simulink model "Model_Platform"  (R2018a)
settings: Solver=ode1  StartTime=0.0  StopTime=inf  FixedStep=0.001  RelTol=1e-3  EnableMultiTasking=on
PreLoadFcn:
  | ;HLABlocksetInit;;HLABlocksetInit;;HLABlocksetInit;
PostLoadFcn:
  | ;set_param(gcs,'PostCodeGenCommand', 'rtw_defines(buildInfo)');;set_param(gcs,'PostCodeGenCommand', 'rtw_defines(buildInfo)');;set_param(gcs,'PostCodeGenCommand', 'rtw_defines(buildInfo)');
undefined symbols (not defined in the file or in its folder): eng_speed, Heading_init, inertiaLateral, Joystick, Newton, omega_engine, omega_max, omega_wheel, Para, radiusWheel, Raphson, Standard_Devices, torque, Torque_lost, Torque_lost_wheel, X_init, Y_init, Z_init
libraries: simulink x26, dspnetwork x4, rtwinlib x2, PC_Simulator_Lib x2, vrlib x1
(part 3 of 4)

== system Model_Platform/Vehicle model/Drive_Train/4_Wheels_drive_train_and_Brake/Brake/Subsystem ==
  Torque_Brake_Nm : Inport
  Omega_rad/s : Inport  Port=2
  Compare To Constant : simulink/Logic and Bit Operations/Compare To Constant  relop=>=  const=0.1  OutDataTypeStr=uint8
  Compare To Constant1 : simulink/Logic and Bit Operations/Compare To Constant  relop=<=  const=-0.1  OutDataTypeStr=uint8
  Data Type Conversion : DataTypeConversion
  Logical Operator : Logic  Operator=OR  AllPortsSameDT=off  OutDataTypeStr=boolean
  Product : Product  Inputs=3  RndMeth=Zero
  Rate Limiter1 : RateLimiter  SampleTimeMode=inherited
  Sign : Signum
  Torque_Brake_act_Nm : Outport
  wires:
  Torque_Brake_Nm/1 -> Product/1
  Omega_rad/s/1 -> Compare To Constant1/1, Compare To Constant/1, Sign/1
  Product/1 -> Torque_Brake_act_Nm/1
  Sign/1 -> Product/2
  Compare To Constant/1 -> Logical Operator/1
  Data Type Conversion/1 -> Rate Limiter1/1
  Logical Operator/1 -> Data Type Conversion/1
  Compare To Constant1/1 -> Logical Operator/2
  Rate Limiter1/1 -> Product/3

== system Model_Platform/Vehicle model/Drive_Train/4_Wheels_drive_train_and_Brake/Brake/Subsystem1 ==
  v_X_CoG[m|s] : Inport
  Brake_Pedal[norm] : Inport  Port=2
  Compare To Constant : simulink/Logic and Bit Operations/Compare To Constant  relop=<  const=0.7  OutDataTypeStr=uint8
  Compare To Constant1 : simulink/Logic and Bit Operations/Compare To Constant  relop=>  const=-1  OutDataTypeStr=uint8
  Compare To Constant2 : simulink/Logic and Bit Operations/Compare To Constant  relop=>=  const=0.01  OutDataTypeStr=uint8
  Compare To Constant3 : simulink/Logic and Bit Operations/Compare To Constant  relop=<  const=-0.1  OutDataTypeStr=uint8
  Constant : Constant  Value=0
  Constant1 : Constant  Value=3.5
  Constant2 : Constant
  Data Type Conversion : DataTypeConversion
  Gain1 : Gain  Gain=-100
  Logical Operator : Logic  Inputs=3  AllPortsSameDT=off  OutDataTypeStr=boolean
  Logical Operator1 : Logic  AllPortsSameDT=off  OutDataTypeStr=boolean
  Product : Product  Inputs=3
  Subtract : Sum  Inputs=+-
  Switch : Switch  Criteria=u2 > Threshold
  Out1 : Outport
  wires:
  Constant2/1 -> Switch/3
  Switch/1 -> Product/3
  Constant1/1 -> Switch/1
  Logical Operator1/1 -> Switch/2
  Compare To Constant3/1 -> Logical Operator1/2
  Brake_Pedal[norm]/1 -> Compare To Constant2/1
  Compare To Constant2/1 -> Logical Operator/3
  Data Type Conversion/1 -> Product/2
  Logical Operator/1 -> Data Type Conversion/1
  Compare To Constant1/1 -> Logical Operator/2, Logical Operator1/1
  Compare To Constant/1 -> Logical Operator/1
  Product/1 -> Out1/1
  Gain1/1 -> Product/1
  Subtract/1 -> Gain1/1
  Constant/1 -> Subtract/1
  v_X_CoG[m|s]/1 -> Subtract/2, Compare To Constant/1, Compare To Constant1/1, Compare To Constant3/1

== system Model_Platform/Vehicle model/Drive_Train/4_Wheels_drive_train_and_Brake/FL/Alpha_Kappa_Selector2 ==
  Vx : Inport
  Vy : Inport  Port=2
  omega : Inport  Port=3
  Rdyn : Inport  Port=4
  Fx : Inport  Port=5
  Dynamik Anteil2 : Subsystem
  Saturation : Saturate  UpperLimit=1  LowerLimit=-1
  alpha_calc : Subsystem
  kappa : Outport
  alpha : Outport  Port=2
  wires:
  Vy/1 -> alpha_calc/1(Vy)
  Vx/1 -> Dynamik Anteil2/2(Vx), alpha_calc/2(Vx)
  alpha_calc/1(alpha) -> alpha/1
  omega/1 -> Dynamik Anteil2/3(omega)
  Rdyn/1 -> Dynamik Anteil2/4(R)
  Saturation/1 -> kappa/1
  Dynamik Anteil2/1(k) -> Saturation/1
  Fx/1 -> Dynamik Anteil2/1(Fx)

== system Model_Platform/Vehicle model/Drive_Train/4_Wheels_drive_train_and_Brake/FL/Wheel dynamics ==
  F_x : Inport
  Torque_Drive_Nm : Inport  Port=2
  Torque_Brake_Nm : Inport  Port=3
  Add : Sum  Inputs=++--
  Friction : Subsystem
  Gain : Gain  Gain=radiusWheel
  Gain1 : Gain  Gain=-1
  Gain2 : Gain  Gain=1/(inertiaLateral/2)
  Integrator : Integrator
  Subsystem : Subsystem
  Terminator : Terminator
  omega_radPs : Outport
  omegaDot_radPs2 : Outport  Port=2
  wires:
  Subsystem/1(Torque_Brake_act_Nm) -> Terminator/1
  Torque_Brake_Nm/1 -> Add/4, Subsystem/1(Torque_Brake_Nm)
  Friction/1(Torque_friction) -> Add/3
  Integrator/1 -> Subsystem/2(Omega_rad/s), Friction/1(omega_radPs), omega_radPs/1
  Gain2/1 -> omegaDot_radPs2/1, Integrator/1
  Add/1 -> Gain2/1
  Torque_Drive_Nm/1 -> Add/2
  Gain1/1 -> Add/1
  F_x/1 -> Gain/1
  Gain/1 -> Gain1/1

== system Model_Platform/Vehicle model/Drive_Train/4_Wheels_drive_train_and_Brake/FR/Alpha_Kappa_Selector2 ==
  Vx : Inport
  Vy : Inport  Port=2
  omega : Inport  Port=3
  Rdyn : Inport  Port=4
  Fx : Inport  Port=5
  Dynamik Anteil2 : Subsystem
  Saturation : Saturate  UpperLimit=1  LowerLimit=-1
  alpha_calc : Subsystem
  kappa : Outport
  alpha : Outport  Port=2
  wires:
  Vy/1 -> alpha_calc/1(Vy)
  Vx/1 -> Dynamik Anteil2/2(Vx), alpha_calc/2(Vx)
  alpha_calc/1(alpha) -> alpha/1
  omega/1 -> Dynamik Anteil2/3(omega)
  Rdyn/1 -> Dynamik Anteil2/4(R)
  Saturation/1 -> kappa/1
  Dynamik Anteil2/1(k) -> Saturation/1
  Fx/1 -> Dynamik Anteil2/1(Fx)

== system Model_Platform/Vehicle model/Drive_Train/4_Wheels_drive_train_and_Brake/FR/Wheel dynamics ==
  F_x : Inport
  Torque_Drive_Nm : Inport  Port=2
  Torque_Brake_Nm : Inport  Port=3
  Add : Sum  Inputs=++--
  Friction : Subsystem
  Gain : Gain  Gain=radiusWheel
  Gain1 : Gain  Gain=-1
  Gain2 : Gain  Gain=1/(inertiaLateral/2)
  Integrator : Integrator
  Subsystem : Subsystem
  Terminator : Terminator
  omega_radPs : Outport
  omegaDot_radPs2 : Outport  Port=2
  wires:
  Subsystem/1(Torque_Brake_act_Nm) -> Terminator/1
  Torque_Brake_Nm/1 -> Add/4, Subsystem/1(Torque_Brake_Nm)
  Friction/1(Torque_friction) -> Add/3
  Integrator/1 -> Subsystem/2(Omega_rad/s), Friction/1(omega_radPs), omega_radPs/1
  Gain2/1 -> omegaDot_radPs2/1, Integrator/1
  Add/1 -> Gain2/1
  Torque_Drive_Nm/1 -> Add/2
  Gain1/1 -> Add/1
  F_x/1 -> Gain/1
  Gain/1 -> Gain1/1

== system Model_Platform/Vehicle model/Drive_Train/4_Wheels_drive_train_and_Brake/RL/Alpha_Kappa_Selector2 ==
  Vx : Inport
  Vy : Inport  Port=2
  omega : Inport  Port=3
  Rdyn : Inport  Port=4
  Fx : Inport  Port=5
  Dynamik Anteil2 : Subsystem
  Saturation : Saturate  UpperLimit=1  LowerLimit=-1
  alpha_calc : Subsystem
  kappa : Outport
  alpha : Outport  Port=2
  wires:
  Vy/1 -> alpha_calc/1(Vy)
  Vx/1 -> Dynamik Anteil2/2(Vx), alpha_calc/2(Vx)
  alpha_calc/1(alpha) -> alpha/1
  omega/1 -> Dynamik Anteil2/3(omega)
  Rdyn/1 -> Dynamik Anteil2/4(R)
  Saturation/1 -> kappa/1
  Dynamik Anteil2/1(k) -> Saturation/1
  Fx/1 -> Dynamik Anteil2/1(Fx)

== system Model_Platform/Vehicle model/Drive_Train/4_Wheels_drive_train_and_Brake/RL/Wheel dynamics ==
  F_x : Inport
  Torque_Drive_Nm : Inport  Port=2
  Torque_Brake_Nm : Inport  Port=3
  Add : Sum  Inputs=++--
  Friction : Subsystem
  Gain : Gain  Gain=radiusWheel
  Gain1 : Gain  Gain=-1
  Gain2 : Gain  Gain=1/(inertiaLateral/2)
  Integrator : Integrator
  Subsystem : Subsystem
  Terminator : Terminator
  omega_radPs : Outport
  omegaDot_radPs2 : Outport  Port=2
  wires:
  Subsystem/1(Torque_Brake_act_Nm) -> Terminator/1
  Torque_Brake_Nm/1 -> Add/4, Subsystem/1(Torque_Brake_Nm)
  Friction/1(Torque_friction) -> Add/3
  Integrator/1 -> Subsystem/2(Omega_rad/s), Friction/1(omega_radPs), omega_radPs/1
  Gain2/1 -> omegaDot_radPs2/1, Integrator/1
  Add/1 -> Gain2/1
  Torque_Drive_Nm/1 -> Add/2
  Gain1/1 -> Add/1
  F_x/1 -> Gain/1
  Gain/1 -> Gain1/1

== system Model_Platform/Vehicle model/Drive_Train/4_Wheels_drive_train_and_Brake/RR/Alpha_Kappa_Selector2 ==
  Vx : Inport
  Vy : Inport  Port=2
  omega : Inport  Port=3
  Rdyn : Inport  Port=4
  Fx : Inport  Port=5
  Dynamik Anteil2 : Subsystem
  Saturation : Saturate  UpperLimit=1  LowerLimit=-1
  alpha_calc : Subsystem
  kappa : Outport
  alpha : Outport  Port=2
  wires:
  Vy/1 -> alpha_calc/1(Vy)
  Vx/1 -> Dynamik Anteil2/2(Vx), alpha_calc/2(Vx)
  alpha_calc/1(alpha) -> alpha/1
  omega/1 -> Dynamik Anteil2/3(omega)
  Rdyn/1 -> Dynamik Anteil2/4(R)
  Saturation/1 -> kappa/1
  Dynamik Anteil2/1(k) -> Saturation/1
  Fx/1 -> Dynamik Anteil2/1(Fx)

== system Model_Platform/Vehicle model/Drive_Train/4_Wheels_drive_train_and_Brake/RR/Wheel dynamics ==
  F_x : Inport
  Torque_Drive_Nm : Inport  Port=2
  Torque_Brake_Nm : Inport  Port=3
  Add : Sum  Inputs=++--
  Friction : Subsystem
  Gain : Gain  Gain=radiusWheel
  Gain1 : Gain  Gain=-1
  Gain2 : Gain  Gain=1/(inertiaLateral/2)
  Integrator : Integrator
  Subsystem : Subsystem
  Terminator : Terminator
  omega_radPs : Outport
  omegaDot_radPs2 : Outport  Port=2
  wires:
  Subsystem/1(Torque_Brake_act_Nm) -> Terminator/1
  Torque_Brake_Nm/1 -> Add/4, Subsystem/1(Torque_Brake_Nm)
  Friction/1(Torque_friction) -> Add/3
  Integrator/1 -> Subsystem/2(Omega_rad/s), Friction/1(omega_radPs), omega_radPs/1
  Gain2/1 -> omegaDot_radPs2/1, Integrator/1
  Add/1 -> Gain2/1
  Torque_Drive_Nm/1 -> Add/2
  Gain1/1 -> Add/1
  F_x/1 -> Gain/1
  Gain/1 -> Gain1/1

== system Model_Platform/Vehicle model/Vehicle dynamics/Vertical_Dyn./suspention_System/Rear_Right_Suspention ==
  note: Vertical_Velocity_Z_vehicle_corner_RR
  note: Spring_intial_length+Spring_precompressed_length = Spring_Free_length
  note: U
  note: Fs=K(Lf-(L0 - U))
  note: Fs=f0s+KU
  Vertical_Displacement_Z_vehicle_corner_RR : Inport
  Vertical_Displacement_Z0 : Inport  Port=2
  intial_force_form_mass_rr : Inport  Port=3
  Add1 : Sum  Inputs=+++
  Add2 : Sum  Inputs=+-
  Constant : Constant  Value=0
  Constant2 : Constant  Value=Para.VD.Spring_intial_length.v
  Gain : Gain  Gain=Para.VD.Spring_Stifness_Rear.v
  Gain2 : Gain  Gain=Para.VD.Damper_Damping_Constant_Rear.v
  Relational Operator : RelationalOperator  Operator=>  OutDataTypeStr=boolean  ZeroCross=off  RndMeth=Nearest
  Relational Operator1 : RelationalOperator  Operator=<  OutDataTypeStr=boolean  ZeroCross=off  RndMeth=Nearest
  Saturation : Saturate  UpperLimit=Para.VD.Spring_intial_length.v-Para.VD.Spring_Lower_limit.v  LowerLimit=Para.VD.Spring_intial_length.v-Para.VD.Spring_Upper_limit.v
  Subtract : Sum  Inputs=+-
  Subtract1 : Sum  Inputs=+-
  Subtract2 : Sum  Inputs=+-
  Switch : Switch
  Switch1 : Switch
  Transfer Fcn : TransferFcn  Numerator=[1 0]  Denominator=[0.001 1]
  vertical_dynamics_tire : Subsystem
  Force_Suspention_RR : Outport
  Hight_Reer_Right : Outport  Port=2
  Z1 : Outport  Port=3
  Z2actual : Outport  Port=4
  wires:
  Relational Operator1/1 -> Switch1/2
  Switch1/1 -> Add1/3
  Constant/1 -> Switch1/1
  Switch/1 -> Z2actual/1
  Relational Operator/1 -> Switch/2
  Add2/1 -> Switch/1
  intial_force_form_mass_rr/1 -> Switch1/3, vertical_dynamics_tire/3(intial_force_form_mass)
  vertical_dynamics_tire/2(Vertical_Velocity_Z1_Wheel) -> Subtract1/1
  Vertical_Displacement_Z0/1 -> vertical_dynamics_tire/2(Vertical_Displacement_Z0_Road)
  vertical_dynamics_tire/1(Vertical_Displacement_Z1_Wheel) -> Add2/1, Z1/1, Subtract/1
  Gain/1 -> Add1/1
  Subtract1/1 -> Gain2/1
  Gain2/1 -> Add1/2
  Add1/1 -> vertical_dynamics_tire/1(Force_Suspention), Force_Suspention_RR/1
  Saturation/1 -> Relational Operator1/2, Relational Operator/2, Add2/2, Subtract2/2, Gain/1
  Subtract/1 -> Relational Operator1/1, Relational Operator/1, Saturation/1
  Vertical_Displacement_Z_vehicle_corner_RR/1 -> Switch/3, Transfer Fcn/1, Subtract/2
  Transfer Fcn/1 -> Subtract1/2
  Constant2/1 -> Subtract2/1
  Subtract2/1 -> Hight_Reer_Right/1

== system Model_Platform/Vehicle model/Vehicle dynamics/Vertical_Dyn./suspention_System/Rear_left_Suspention ==
  note: Fs=f0s+KU
  note: Fs=K(Lf-(L0 - U))
  note: U
  note: Spring_intial_length+Spring_precompressed_length = Spring_Free_length
  note: Vertical_Velocity_Z_vehicle_corner_RR
  Vertical_Displacement_Z_vehicle_corner_Rl : Inport
  Vertical_Displacement_Z0 : Inport  Port=2
  intial_force_form_mass_rl : Inport  Port=3
  Add1 : Sum  Inputs=+++
  Add2 : Sum  Inputs=+-
  Constant : Constant  Value=0
  Constant2 : Constant  Value=Para.VD.Spring_intial_length.v
  Gain : Gain  Gain=Para.VD.Spring_Stifness_Rear.v
  Gain2 : Gain  Gain=Para.VD.Damper_Damping_Constant_Rear.v
  Relational Operator : RelationalOperator  Operator=>  OutDataTypeStr=boolean  ZeroCross=off  RndMeth=Nearest
  Relational Operator1 : RelationalOperator  Operator=<  OutDataTypeStr=boolean  ZeroCross=off  RndMeth=Nearest
  Saturation : Saturate  UpperLimit=Para.VD.Spring_intial_length.v-Para.VD.Spring_Lower_limit.v  LowerLimit=Para.VD.Spring_intial_length.v-Para.VD.Spring_Upper_limit.v
  Subtract : Sum  Inputs=+-
  Subtract1 : Sum  Inputs=+-
  Subtract2 : Sum  Inputs=+-
  Switch : Switch
  Switch1 : Switch
  Transfer Fcn : TransferFcn  Numerator=[1 0]  Denominator=[0.001 1]
  vertical_dynamics_tire : Subsystem
  Force_Suspention_RL : Outport
  Hight_Reer_left : Outport  Port=2
  Z1 : Outport  Port=3
  Z2actual : Outport  Port=4
  wires:
  Relational Operator1/1 -> Switch1/2
  Switch1/1 -> Add1/3
  Constant/1 -> Switch1/1
  Switch/1 -> Z2actual/1
  Relational Operator/1 -> Switch/2
  Add2/1 -> Switch/1
  Subtract2/1 -> Hight_Reer_left/1
  Constant2/1 -> Subtract2/1
  Transfer Fcn/1 -> Subtract1/2
  Vertical_Displacement_Z_vehicle_corner_Rl/1 -> Subtract/2, Transfer Fcn/1, Switch/3
  Subtract/1 -> Relational Operator1/1, Relational Operator/1, Saturation/1
  Saturation/1 -> Relational Operator1/2, Add2/2, Subtract2/2, Relational Operator/2, Gain/1
  Add1/1 -> Force_Suspention_RL/1, vertical_dynamics_tire/1(Force_Suspention)
  Gain2/1 -> Add1/2
  Subtract1/1 -> Gain2/1
  Gain/1 -> Add1/1
  vertical_dynamics_tire/1(Vertical_Displacement_Z1_Wheel) -> Add2/1, Z1/1, Subtract/1
  Vertical_Displacement_Z0/1 -> vertical_dynamics_tire/2(Vertical_Displacement_Z0_Road)
  vertical_dynamics_tire/2(Vertical_Velocity_Z1_Wheel) -> Subtract1/1
  intial_force_form_mass_rl/1 -> Switch1/3, vertical_dynamics_tire/3(intial_force_form_mass)

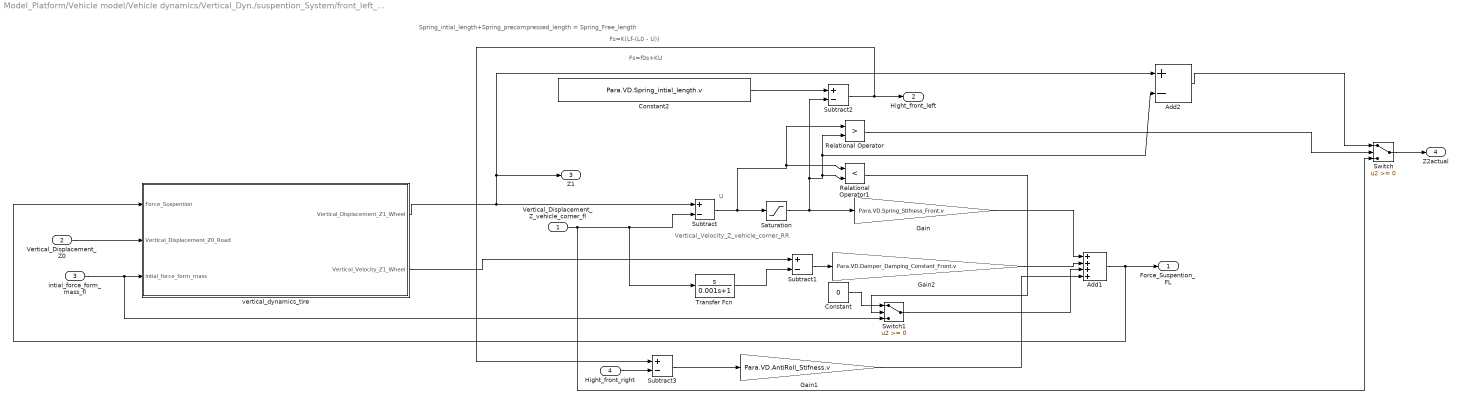
== system Model_Platform/Vehicle model/Vehicle dynamics/Vertical_Dyn./suspention_System/front_left_Suspention ==
  note: Vertical_Velocity_Z_vehicle_corner_RR
  note: Spring_intial_length+Spring_precompressed_length = Spring_Free_length
  note: U
  note: Fs=K(Lf-(L0 - U))
  note: Fs=f0s+KU
  Vertical_Displacement_Z_vehicle_corner_fl : Inport
  Vertical_Displacement_Z0 : Inport  Port=2
  intial_force_form_mass_fl : Inport  Port=3
  Hight_front_right : Inport  Port=4
  Add1 : Sum  Inputs=++++
  Add2 : Sum  Inputs=+-
  Constant : Constant  Value=0
  Constant2 : Constant  Value=Para.VD.Spring_intial_length.v
  Gain : Gain  Gain=Para.VD.Spring_Stifness_Front.v
  Gain1 : Gain  Gain=Para.VD.AntiRoll_Stifness.v
  Gain2 : Gain  Gain=Para.VD.Damper_Damping_Constant_Front.v
  Relational Operator : RelationalOperator  Operator=>  OutDataTypeStr=boolean  ZeroCross=off  RndMeth=Nearest
  Relational Operator1 : RelationalOperator  Operator=<  OutDataTypeStr=boolean  ZeroCross=off  RndMeth=Nearest
  Saturation : Saturate  UpperLimit=Para.VD.Spring_intial_length.v-Para.VD.Spring_Lower_limit.v  LowerLimit=Para.VD.Spring_intial_length.v-Para.VD.Spring_Upper_limit.v  ZeroCross=off
  Subtract{,1..3} (4 alike) : Sum  Inputs=+-
  Switch : Switch
  Switch1 : Switch
  Transfer Fcn : TransferFcn  Numerator=[1 0]  Denominator=[0.001 1]
  vertical_dynamics_tire : Subsystem
  Force_Suspention_FL : Outport
  Hight_front_left : Outport  Port=2
  Z1 : Outport  Port=3
  Z2actual : Outport  Port=4
  wires:
  Relational Operator1/1 -> Switch1/2
  Switch1/1 -> Add1/3
  Constant/1 -> Switch1/1
  Gain1/1 -> Add1/4
  Subtract3/1 -> Gain1/1
  Hight_front_right/1 -> Subtract3/2
  Switch/1 -> Z2actual/1
  Relational Operator/1 -> Switch/2
  Add2/1 -> Switch/1
  intial_force_form_mass_fl/1 -> Switch1/3, vertical_dynamics_tire/3(intial_force_form_mass)
  vertical_dynamics_tire/2(Vertical_Velocity_Z1_Wheel) -> Subtract1/1
  Vertical_Displacement_Z0/1 -> vertical_dynamics_tire/2(Vertical_Displacement_Z0_Road)
  vertical_dynamics_tire/1(Vertical_Displacement_Z1_Wheel) -> Add2/1, Z1/1, Subtract/1
  Gain/1 -> Add1/1
  Subtract1/1 -> Gain2/1
  Gain2/1 -> Add1/2
  Add1/1 -> Force_Suspention_FL/1, vertical_dynamics_tire/1(Force_Suspention)
  Saturation/1 -> Gain/1, Relational Operator1/2, Add2/2, Relational Operator/2, Subtract2/2
  Subtract/1 -> Relational Operator1/1, Relational Operator/1, Saturation/1
  Vertical_Displacement_Z_vehicle_corner_fl/1 -> Switch/3, Transfer Fcn/1, Subtract/2
  Transfer Fcn/1 -> Subtract1/2
  Constant2/1 -> Subtract2/1
  Subtract2/1 -> Subtract3/1, Hight_front_left/1

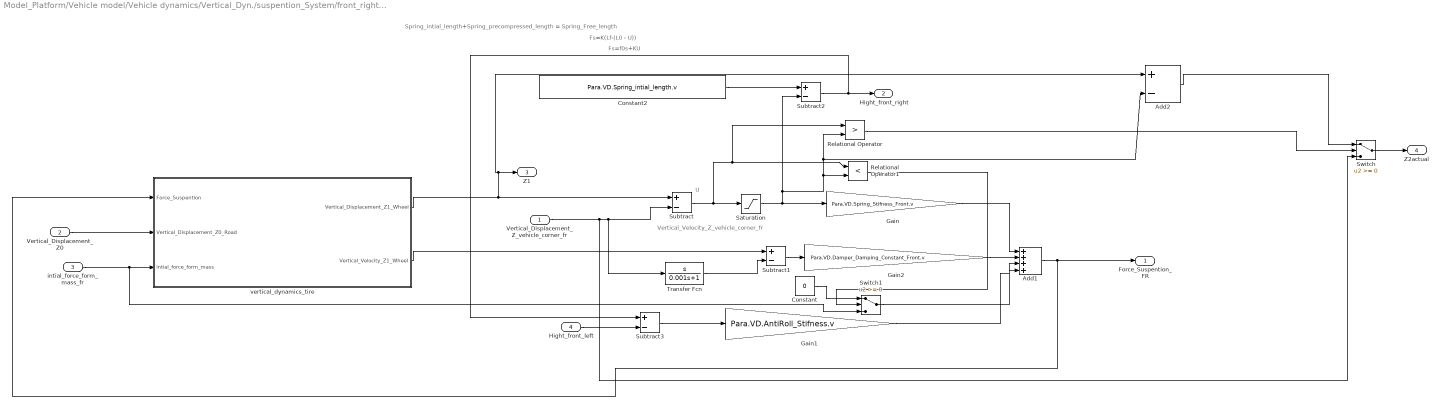
== system Model_Platform/Vehicle model/Vehicle dynamics/Vertical_Dyn./suspention_System/front_right_Suspention ==
  note: Fs=f0s+KU
  note: Fs=K(Lf-(L0 - U))
  note: U
  note: Spring_intial_length+Spring_precompressed_length = Spring_Free_length
  note: Vertical_Velocity_Z_vehicle_corner_fr
  Vertical_Displacement_Z_vehicle_corner_fr : Inport
  Vertical_Displacement_Z0 : Inport  Port=2
  intial_force_form_mass_fr : Inport  Port=3
  Hight_front_left : Inport  Port=4
  Add1 : Sum  Inputs=++++
  Add2 : Sum  Inputs=+-
  Constant : Constant  Value=0
  Constant2 : Constant  Value=Para.VD.Spring_intial_length.v
  Gain : Gain  Gain=Para.VD.Spring_Stifness_Front.v
  Gain1 : Gain  Gain=Para.VD.AntiRoll_Stifness.v
  Gain2 : Gain  Gain=Para.VD.Damper_Damping_Constant_Front.v
  Relational Operator : RelationalOperator  Operator=>  OutDataTypeStr=boolean  ZeroCross=off  RndMeth=Nearest
  Relational Operator1 : RelationalOperator  Operator=<  OutDataTypeStr=boolean  ZeroCross=off  RndMeth=Nearest
  Saturation : Saturate  UpperLimit=Para.VD.Spring_intial_length.v-Para.VD.Spring_Lower_limit.v  LowerLimit=Para.VD.Spring_intial_length.v-Para.VD.Spring_Upper_limit.v
  Subtract{,1..3} (4 alike) : Sum  Inputs=+-
  Switch : Switch
  Switch1 : Switch
  Transfer Fcn : TransferFcn  Numerator=[1 0]  Denominator=[0.001 1]
  vertical_dynamics_tire : Subsystem
  Force_Suspention_FR : Outport
  Hight_front_right : Outport  Port=2
  Z1 : Outport  Port=3
  Z2actual : Outport  Port=4
  wires:
  Relational Operator1/1 -> Switch1/2
  Switch1/1 -> Add1/3
  Constant/1 -> Switch1/1
  Hight_front_left/1 -> Subtract3/2
  Subtract3/1 -> Gain1/1
  Gain1/1 -> Add1/4
  Switch/1 -> Z2actual/1
  Relational Operator/1 -> Switch/2
  Add2/1 -> Switch/1
  Subtract2/1 -> Subtract3/1, Hight_front_right/1
  Constant2/1 -> Subtract2/1
  Transfer Fcn/1 -> Subtract1/2
  Vertical_Displacement_Z_vehicle_corner_fr/1 -> Switch/3, Transfer Fcn/1, Subtract/2
  Subtract/1 -> Relational Operator1/1, Relational Operator/1, Saturation/1
  Saturation/1 -> Relational Operator1/2, Add2/2, Relational Operator/2, Subtract2/2, Gain/1
  Add1/1 -> Force_Suspention_FR/1, vertical_dynamics_tire/1(Force_Suspention)
  Gain2/1 -> Add1/2
  Subtract1/1 -> Gain2/1
  Gain/1 -> Add1/1
  vertical_dynamics_tire/1(Vertical_Displacement_Z1_Wheel) -> Add2/1, Z1/1, Subtract/1
  Vertical_Displacement_Z0/1 -> vertical_dynamics_tire/2(Vertical_Displacement_Z0_Road)
  vertical_dynamics_tire/2(Vertical_Velocity_Z1_Wheel) -> Subtract1/1
  intial_force_form_mass_fr/1 -> Switch1/3, vertical_dynamics_tire/3(intial_force_form_mass)

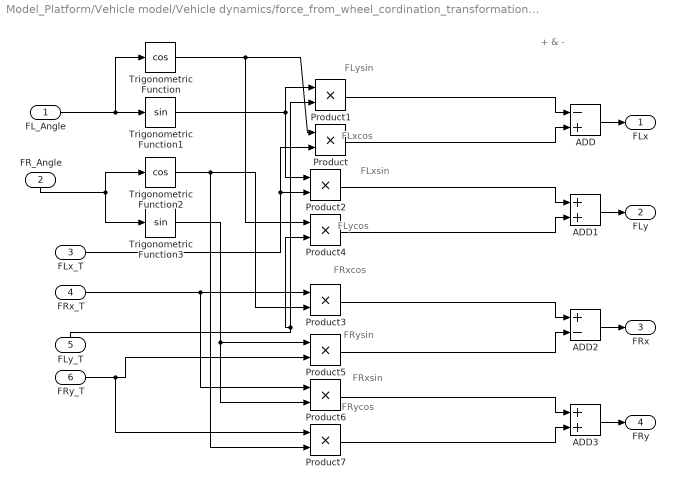
== system Model_Platform/Vehicle model/Vehicle dynamics/force_from_wheel_cordination_transformation/Steer_model/Force_Analysis ==
  note: + & -
  note: FRycos
  note: FRxsin
  note: FRysin
  note: FRxcos
  note: FLycos
  note: FLxsin
  note: FLxcos
  note: FLysin
  FL_Angle : Inport
  FR_Angle : Inport  Port=2
  FLx_T : Inport  Port=3
  FRx_T : Inport  Port=4
  FLy_T : Inport  Port=5
  FRy_T : Inport  Port=6
  ADD : Sum  Inputs=-+
  ADD1 : Sum
  ADD2 : Sum  Inputs=+-
  ADD3 : Sum
  Product{,1..7} (8 alike) : Product  RndMeth=Zero
  Trigonometric Function : Trigonometry  Operator=cos
  Trigonometric Function1 : Trigonometry
  Trigonometric Function2 : Trigonometry  Operator=cos
  Trigonometric Function3 : Trigonometry
  FLx : Outport
  FLy : Outport  Port=2
  FRx : Outport  Port=3
  FRy : Outport  Port=4
  wires:
  Trigonometric Function3/1 -> Product6/2, Product5/1
  ADD3/1 -> FRy/1
  ADD2/1 -> FRx/1
  ADD1/1 -> FLy/1
  ADD/1 -> FLx/1
  Product7/1 -> ADD3/2
  Product6/1 -> ADD3/1
  Product5/1 -> ADD2/2
  FRy_T/1 -> Product7/1, Product5/2
  Product3/1 -> ADD2/1
  Trigonometric Function2/1 -> Product7/2, Product3/2
  FRx_T/1 -> Product6/1, Product3/1
  Product4/1 -> ADD1/2
  Product2/1 -> ADD1/1
  Product1/1 -> ADD/1
  Trigonometric Function1/1 -> Product2/1, Product1/1
  FLy_T/1 -> Product4/2, Product1/2
  FLx_T/1 -> Product/2, Product2/2
  Product/1 -> ADD/2
  Trigonometric Function/1 -> Product/1, Product4/1
  FR_Angle/1 -> Trigonometric Function3/1, Trigonometric Function2/1
  FL_Angle/1 -> Trigonometric Function1/1, Trigonometric Function/1

== system Model_Platform/Vehicle model/Vehicle dynamics/force_from_wheel_cordination_transformation/Steer_model/Steer_Angel_Distribution1 ==
  note: Turning_Radius_Measured_From_The_Edge
  Steering_Angle_HMI_[-1 1] : Inport
  Divide : Product  Inputs=*/
  Divide1 : Product  Inputs=*/
  Divide2 : Product  Inputs=*/
  Gain1 : Gain  Gain=0.5
  Gain2 : Gain  Gain=2
  Minimum_Turning_Radius : Constant  Value=Para.VD.Minimum_Turning_Radius.v
  Sum : Sum  Inputs=|+-
  Sum1 : Sum  Inputs=|++
  Trigonometric Function : Trigonometry  Operator=atan
  Trigonometric Function1 : Trigonometry  Operator=atan
  Wheel_Base_Length : Constant  Value=Para.VD.Wheel_Base_Length.v
  Wheel_Base_Width : Constant  Value=Para.VD.Wheel_Base_Width.v
  FL_Angle : Outport
  FR_Angle : Outport  Port=2
  wires:
  Steering_Angle_HMI_[-1 1]/1 -> Gain2/1
  Trigonometric Function1/1 -> FR_Angle/1
  Trigonometric Function/1 -> FL_Angle/1
  Gain2/1 -> Divide/2
  Gain1/1 -> Sum1/2, Sum/2
  Sum1/1 -> Divide2/2
  Sum/1 -> Divide1/2
  Divide2/1 -> Trigonometric Function1/1
  Divide1/1 -> Trigonometric Function/1
  Wheel_Base_Length/1 -> Divide2/1, Divide1/1
  Wheel_Base_Width/1 -> Gain1/1
  Divide/1 -> Sum1/1, Sum/1
  Minimum_Turning_Radius/1 -> Divide/1

== system Model_Platform/Vehicle model/Vehicle dynamics/velocity/velocity_conditioning/Velocitytrim ==
  vin : Inport
  Abs : Abs
  Constant2 : Constant  Value=0
  Constant6 : Constant  Value=10*eps
  Relational Operator3 : RelationalOperator  Operator=>  OutDataTypeStr=boolean  RndMeth=Nearest
  Switch4 : Switch
  vout : Outport
  wires:
  Switch4/1 -> vout/1
  vin/1 -> Switch4/1, Abs/1
  Relational Operator3/1 -> Switch4/2
  Constant2/1 -> Switch4/3
  Constant6/1 -> Relational Operator3/2
  Abs/1 -> Relational Operator3/1

== system Model_Platform/Vehicle model/Vehicle dynamics/velocity/velocity_conditioning/Velocitytrim1 ==
  vin : Inport
  Abs : Abs
  Constant2 : Constant  Value=0
  Constant6 : Constant  Value=10*eps
  Relational Operator3 : RelationalOperator  Operator=>  OutDataTypeStr=boolean  RndMeth=Nearest
  Switch4 : Switch
  vout : Outport
  wires:
  Abs/1 -> Relational Operator3/1
  Constant6/1 -> Relational Operator3/2
  Constant2/1 -> Switch4/3
  Relational Operator3/1 -> Switch4/2
  vin/1 -> Abs/1, Switch4/1
  Switch4/1 -> vout/1

== system Model_Platform/Vehicle model/Vehicle dynamics/velocity/velocity_conditioning/Velocitytrim2 ==
  vin : Inport
  Abs : Abs
  Constant2 : Constant  Value=0
  Constant6 : Constant  Value=10*eps
  Relational Operator3 : RelationalOperator  Operator=>  OutDataTypeStr=boolean  RndMeth=Nearest
  Switch4 : Switch
  vout : Outport
  wires:
  Switch4/1 -> vout/1
  vin/1 -> Switch4/1, Abs/1
  Relational Operator3/1 -> Switch4/2
  Constant2/1 -> Switch4/3
  Constant6/1 -> Relational Operator3/2
  Abs/1 -> Relational Operator3/1

== system Model_Platform/Vehicle model/Vehicle dynamics/velocity/velocity_conditioning/Velocitytrim3 ==
  vin : Inport
  Abs : Abs
  Constant2 : Constant  Value=0
  Constant6 : Constant  Value=10*eps
  Relational Operator3 : RelationalOperator  Operator=>  OutDataTypeStr=boolean  RndMeth=Nearest
  Switch4 : Switch
  vout : Outport
  wires:
  Abs/1 -> Relational Operator3/1
  Constant6/1 -> Relational Operator3/2
  Constant2/1 -> Switch4/3
  Relational Operator3/1 -> Switch4/2
  vin/1 -> Abs/1, Switch4/1
  Switch4/1 -> vout/1

== system Model_Platform/Vehicle model/Vehicle dynamics/velocity/velocity_conditioning/Velocitytrim4 ==
  vin : Inport
  Abs : Abs
  Constant2 : Constant  Value=0
  Constant6 : Constant  Value=10*eps
  Relational Operator3 : RelationalOperator  Operator=>  OutDataTypeStr=boolean  RndMeth=Nearest
  Switch4 : Switch
  vout : Outport
  wires:
  Abs/1 -> Relational Operator3/1
  Constant6/1 -> Relational Operator3/2
  Constant2/1 -> Switch4/3
  Relational Operator3/1 -> Switch4/2
  vin/1 -> Abs/1, Switch4/1
  Switch4/1 -> vout/1

== system Model_Platform/Vehicle model/Vehicle dynamics/velocity/velocity_conditioning/Velocitytrim5 ==
  vin : Inport
  Abs : Abs
  Constant2 : Constant  Value=0
  Constant6 : Constant  Value=10*eps
  Relational Operator3 : RelationalOperator  Operator=>  OutDataTypeStr=boolean  RndMeth=Nearest
  Switch4 : Switch
  vout : Outport
  wires:
  Switch4/1 -> vout/1
  vin/1 -> Switch4/1, Abs/1
  Relational Operator3/1 -> Switch4/2
  Constant2/1 -> Switch4/3
  Constant6/1 -> Relational Operator3/2
  Abs/1 -> Relational Operator3/1

== system Model_Platform/Vehicle model/Vehicle dynamics/velocity/velocity_conditioning/Velocitytrim6 ==
  vin : Inport
  Abs : Abs
  Constant2 : Constant  Value=0
  Constant6 : Constant  Value=10*eps
  Relational Operator3 : RelationalOperator  Operator=>  OutDataTypeStr=boolean  RndMeth=Nearest
  Switch4 : Switch
  vout : Outport
  wires:
  Abs/1 -> Relational Operator3/1
  Constant6/1 -> Relational Operator3/2
  Constant2/1 -> Switch4/3
  Relational Operator3/1 -> Switch4/2
  vin/1 -> Abs/1, Switch4/1
  Switch4/1 -> vout/1

== system Model_Platform/Vehicle model/Vehicle dynamics/velocity/velocity_conditioning/Velocitytrim7 ==
  vin : Inport
  Abs : Abs
  Constant2 : Constant  Value=0
  Constant6 : Constant  Value=10*eps
  Relational Operator3 : RelationalOperator  Operator=>  OutDataTypeStr=boolean  RndMeth=Nearest
  Switch4 : Switch
  vout : Outport
  wires:
  Switch4/1 -> vout/1
  vin/1 -> Switch4/1, Abs/1
  Relational Operator3/1 -> Switch4/2
  Constant2/1 -> Switch4/3
  Constant6/1 -> Relational Operator3/2
  Abs/1 -> Relational Operator3/1

== system Model_Platform/Vehicle model/Drive_Train/4_Wheels_drive_train_and_Brake/FL/Alpha_Kappa_Selector2/Dynamik Anteil2 ==
  Fx : Inport
  Vx : Inport  Port=2
  omega : Inport  Port=3
  R : Inport  Port=4
  Abs : Abs
  Constant : Constant  Value=1000
  Constant1 : Constant  Value=1000
  Constant2 : Constant  Value=100
  Divide1 : Product  Inputs=*/
  Gain2 : Gain  Gain=-1
  Integrator : Integrator
  Integrator1 : Integrator
  Product : Product  RndMeth=Zero
  Product1 : Product  RndMeth=Zero
  Product2 : Product  RndMeth=Zero
  Product5 : Product  Inputs=*/  RndMeth=Zero
  Subsystem3 : Subsystem
  Sum : Sum  Inputs=|+-
  Sum1 : Sum  Inputs=|+-
  Sum2 : Sum  Inputs=|+--
  k : Outport
  wires:
  Product5/1 -> k/1
  Subsystem3/1(Out1) -> Product5/2
  Gain2/1 -> Product5/1
  omega/1 -> Product/1
  Vx/1 -> Sum/1, Abs/1
  Product/1 -> Sum/2
  Sum/1 -> Sum1/2  "Vsx"
  Sum1/1 -> Product1/1, Integrator/1
  Integrator/1 -> Product2/1
  Product2/1 -> Sum2/2
  Product1/1 -> Sum2/3
  Integrator1/1 -> Sum1/1, Gain2/1  "Vsxstern"
  Sum2/1 -> Divide1/1
  Divide1/1 -> Integrator1/1
  Abs/1 -> Subsystem3/1(In1)
  Fx/1 -> Sum2/1
  Constant/1 -> Product1/2  "<dcx>"
  Constant1/1 -> Product2/2  "<kcx>"
  R/1 -> Product/2
  Constant2/1 -> Divide1/2

== system Model_Platform/Vehicle model/Drive_Train/4_Wheels_drive_train_and_Brake/FL/Alpha_Kappa_Selector2/alpha_calc ==
  Vy : Inport
  Vx : Inport  Port=2
  Ground : Ground
  Slip_angle_Calculation_From_Vx_and_Vy1 : Subsystem
  Terminator : Terminator
  front : Subsystem
  alpha : Outport
  wires:
  Slip_angle_Calculation_From_Vx_and_Vy1/1(Slip_Angle[deg]) -> alpha/1
  Ground/1 -> front/3(steering_angle)
  front/1(alpha) -> Terminator/1
  Vy/1 -> front/1(Vy), Slip_angle_Calculation_From_Vx_and_Vy1/2(Vy_CoG[m|s])
  Vx/1 -> front/2(Vx), Slip_angle_Calculation_From_Vx_and_Vy1/1(Vx_CoG[m|s])

== system Model_Platform/Vehicle model/Drive_Train/4_Wheels_drive_train_and_Brake/FL/Wheel dynamics/Friction ==
  omega_radPs : Inport
  Lookup Table : Lookup_n-D  NumberOfTableDimensions=1  BreakpointsForDimension1=omega_wheel  BeginIndexSearchUsingPreviousIndexResult=on  Table=Torque_lost_wheel  InputSameDT=on
  Product : Product  RndMeth=Zero
  Torque_friction : Outport
  wires:
  Lookup Table/1 -> Product/1
  Product/1 -> Torque_friction/1
  omega_radPs/1 -> Lookup Table/1, Product/2

== system Model_Platform/Vehicle model/Drive_Train/4_Wheels_drive_train_and_Brake/FL/Wheel dynamics/Subsystem ==
  Torque_Brake_Nm : Inport
  Omega_rad/s : Inport  Port=2
  Compare To Constant : simulink/Logic and Bit Operations/Compare To Constant  relop=>=  const=0.1  OutDataTypeStr=uint8
  Compare To Constant1 : simulink/Logic and Bit Operations/Compare To Constant  relop=<=  const=-0.1  OutDataTypeStr=uint8
  Data Type Conversion : DataTypeConversion
  Logical Operator : Logic  Operator=OR  AllPortsSameDT=off  OutDataTypeStr=boolean
  Product : Product  Inputs=3  RndMeth=Zero
  Rate Limiter1 : RateLimiter  SampleTimeMode=inherited
  Sign : Signum
  Torque_Brake_act_Nm : Outport
  wires:
  Torque_Brake_Nm/1 -> Product/1
  Omega_rad/s/1 -> Compare To Constant1/1, Compare To Constant/1, Sign/1
  Product/1 -> Torque_Brake_act_Nm/1
  Sign/1 -> Product/2
  Compare To Constant/1 -> Logical Operator/1
  Data Type Conversion/1 -> Rate Limiter1/1
  Logical Operator/1 -> Data Type Conversion/1
  Compare To Constant1/1 -> Logical Operator/2
  Rate Limiter1/1 -> Product/3

== system Model_Platform/Vehicle model/Drive_Train/4_Wheels_drive_train_and_Brake/FR/Alpha_Kappa_Selector2/Dynamik Anteil2 ==
  Fx : Inport
  Vx : Inport  Port=2
  omega : Inport  Port=3
  R : Inport  Port=4
  Abs : Abs
  Constant : Constant  Value=1000
  Constant1 : Constant  Value=1000
  Constant2 : Constant  Value=100
  Divide1 : Product  Inputs=*/
  Gain2 : Gain  Gain=-1
  Integrator : Integrator
  Integrator1 : Integrator
  Product : Product  RndMeth=Zero
  Product1 : Product  RndMeth=Zero
  Product2 : Product  RndMeth=Zero
  Product5 : Product  Inputs=*/  RndMeth=Zero
  Subsystem3 : Subsystem
  Sum : Sum  Inputs=|+-
  Sum1 : Sum  Inputs=|+-
  Sum2 : Sum  Inputs=|+--
  k : Outport
  wires:
  Product5/1 -> k/1
  Subsystem3/1(Out1) -> Product5/2
  Gain2/1 -> Product5/1
  omega/1 -> Product/1
  Vx/1 -> Sum/1, Abs/1
  Product/1 -> Sum/2
  Sum/1 -> Sum1/2  "Vsx"
  Sum1/1 -> Product1/1, Integrator/1
  Integrator/1 -> Product2/1
  Product2/1 -> Sum2/2
  Product1/1 -> Sum2/3
  Integrator1/1 -> Sum1/1, Gain2/1  "Vsxstern"
  Sum2/1 -> Divide1/1
  Divide1/1 -> Integrator1/1
  Abs/1 -> Subsystem3/1(In1)
  Fx/1 -> Sum2/1
  Constant/1 -> Product1/2  "<dcx>"
  Constant1/1 -> Product2/2  "<kcx>"
  R/1 -> Product/2
  Constant2/1 -> Divide1/2

== system Model_Platform/Vehicle model/Drive_Train/4_Wheels_drive_train_and_Brake/FR/Alpha_Kappa_Selector2/alpha_calc ==
  Vy : Inport
  Vx : Inport  Port=2
  Ground : Ground
  Slip_angle_Calculation_From_Vx_and_Vy1 : Subsystem
  Terminator : Terminator
  front : Subsystem
  alpha : Outport
  wires:
  Slip_angle_Calculation_From_Vx_and_Vy1/1(Slip_Angle[deg]) -> alpha/1
  Ground/1 -> front/3(steering_angle)
  front/1(alpha) -> Terminator/1
  Vy/1 -> front/1(Vy), Slip_angle_Calculation_From_Vx_and_Vy1/2(Vy_CoG[m|s])
  Vx/1 -> front/2(Vx), Slip_angle_Calculation_From_Vx_and_Vy1/1(Vx_CoG[m|s])

== system Model_Platform/Vehicle model/Drive_Train/4_Wheels_drive_train_and_Brake/FR/Wheel dynamics/Friction ==
  omega_radPs : Inport
  Lookup Table : Lookup_n-D  NumberOfTableDimensions=1  BreakpointsForDimension1=omega_wheel  BeginIndexSearchUsingPreviousIndexResult=on  Table=Torque_lost_wheel  InputSameDT=on
  Product : Product  RndMeth=Zero
  Torque_friction : Outport
  wires:
  Lookup Table/1 -> Product/1
  Product/1 -> Torque_friction/1
  omega_radPs/1 -> Lookup Table/1, Product/2

== system Model_Platform/Vehicle model/Drive_Train/4_Wheels_drive_train_and_Brake/FR/Wheel dynamics/Subsystem ==
  Torque_Brake_Nm : Inport
  Omega_rad/s : Inport  Port=2
  Compare To Constant : simulink/Logic and Bit Operations/Compare To Constant  relop=>=  const=0.1  OutDataTypeStr=uint8
  Compare To Constant1 : simulink/Logic and Bit Operations/Compare To Constant  relop=<=  const=-0.1  OutDataTypeStr=uint8
  Data Type Conversion : DataTypeConversion
  Logical Operator : Logic  Operator=OR  AllPortsSameDT=off  OutDataTypeStr=boolean
  Product : Product  Inputs=3  RndMeth=Zero
  Rate Limiter1 : RateLimiter  SampleTimeMode=inherited
  Sign : Signum
  Torque_Brake_act_Nm : Outport
  wires:
  Torque_Brake_Nm/1 -> Product/1
  Omega_rad/s/1 -> Compare To Constant1/1, Compare To Constant/1, Sign/1
  Product/1 -> Torque_Brake_act_Nm/1
  Sign/1 -> Product/2
  Compare To Constant/1 -> Logical Operator/1
  Data Type Conversion/1 -> Rate Limiter1/1
  Logical Operator/1 -> Data Type Conversion/1
  Compare To Constant1/1 -> Logical Operator/2
  Rate Limiter1/1 -> Product/3

== system Model_Platform/Vehicle model/Drive_Train/4_Wheels_drive_train_and_Brake/RL/Alpha_Kappa_Selector2/Dynamik Anteil2 ==
  Fx : Inport
  Vx : Inport  Port=2
  omega : Inport  Port=3
  R : Inport  Port=4
  Abs : Abs
  Constant : Constant  Value=1000
  Constant1 : Constant  Value=1000
  Constant2 : Constant  Value=100
  Divide1 : Product  Inputs=*/
  Gain2 : Gain  Gain=-1
  Integrator : Integrator
  Integrator1 : Integrator
  Product : Product  RndMeth=Zero
  Product1 : Product  RndMeth=Zero
  Product2 : Product  RndMeth=Zero
  Product5 : Product  Inputs=*/  RndMeth=Zero
  Subsystem3 : Subsystem
  Sum : Sum  Inputs=|+-
  Sum1 : Sum  Inputs=|+-
  Sum2 : Sum  Inputs=|+--
  k : Outport
  wires:
  Product5/1 -> k/1
  Subsystem3/1(Out1) -> Product5/2
  Gain2/1 -> Product5/1
  omega/1 -> Product/1
  Vx/1 -> Sum/1, Abs/1
  Product/1 -> Sum/2
  Sum/1 -> Sum1/2  "Vsx"
  Sum1/1 -> Product1/1, Integrator/1
  Integrator/1 -> Product2/1
  Product2/1 -> Sum2/2
  Product1/1 -> Sum2/3
  Integrator1/1 -> Sum1/1, Gain2/1  "Vsxstern"
  Sum2/1 -> Divide1/1
  Divide1/1 -> Integrator1/1
  Abs/1 -> Subsystem3/1(In1)
  Fx/1 -> Sum2/1
  Constant/1 -> Product1/2  "<dcx>"
  Constant1/1 -> Product2/2  "<kcx>"
  R/1 -> Product/2
  Constant2/1 -> Divide1/2

== system Model_Platform/Vehicle model/Drive_Train/4_Wheels_drive_train_and_Brake/RL/Alpha_Kappa_Selector2/alpha_calc ==
  Vy : Inport
  Vx : Inport  Port=2
  Ground : Ground
  Slip_angle_Calculation_From_Vx_and_Vy1 : Subsystem
  Terminator : Terminator
  front : Subsystem
  alpha : Outport
  wires:
  Slip_angle_Calculation_From_Vx_and_Vy1/1(Slip_Angle[deg]) -> alpha/1
  Ground/1 -> front/3(steering_angle)
  front/1(alpha) -> Terminator/1
  Vy/1 -> front/1(Vy), Slip_angle_Calculation_From_Vx_and_Vy1/2(Vy_CoG[m|s])
  Vx/1 -> front/2(Vx), Slip_angle_Calculation_From_Vx_and_Vy1/1(Vx_CoG[m|s])

== system Model_Platform/Vehicle model/Drive_Train/4_Wheels_drive_train_and_Brake/RL/Wheel dynamics/Friction ==
  omega_radPs : Inport
  Lookup Table : Lookup_n-D  NumberOfTableDimensions=1  BreakpointsForDimension1=omega_wheel  BeginIndexSearchUsingPreviousIndexResult=on  Table=Torque_lost_wheel  InputSameDT=on
  Product : Product  RndMeth=Zero
  Torque_friction : Outport
  wires:
  Lookup Table/1 -> Product/1
  Product/1 -> Torque_friction/1
  omega_radPs/1 -> Lookup Table/1, Product/2

== system Model_Platform/Vehicle model/Drive_Train/4_Wheels_drive_train_and_Brake/RL/Wheel dynamics/Subsystem ==
  Torque_Brake_Nm : Inport
  Omega_rad/s : Inport  Port=2
  Compare To Constant : simulink/Logic and Bit Operations/Compare To Constant  relop=>=  const=0.1  OutDataTypeStr=uint8
  Compare To Constant1 : simulink/Logic and Bit Operations/Compare To Constant  relop=<=  const=-0.1  OutDataTypeStr=uint8
  Data Type Conversion : DataTypeConversion
  Logical Operator : Logic  Operator=OR  AllPortsSameDT=off  OutDataTypeStr=boolean
  Product : Product  Inputs=3  RndMeth=Zero
  Rate Limiter1 : RateLimiter  SampleTimeMode=inherited
  Sign : Signum
  Torque_Brake_act_Nm : Outport
  wires:
  Torque_Brake_Nm/1 -> Product/1
  Omega_rad/s/1 -> Compare To Constant1/1, Compare To Constant/1, Sign/1
  Product/1 -> Torque_Brake_act_Nm/1
  Sign/1 -> Product/2
  Compare To Constant/1 -> Logical Operator/1
  Data Type Conversion/1 -> Rate Limiter1/1
  Logical Operator/1 -> Data Type Conversion/1
  Compare To Constant1/1 -> Logical Operator/2
  Rate Limiter1/1 -> Product/3

== system Model_Platform/Vehicle model/Drive_Train/4_Wheels_drive_train_and_Brake/RR/Alpha_Kappa_Selector2/Dynamik Anteil2 ==
  Fx : Inport
  Vx : Inport  Port=2
  omega : Inport  Port=3
  R : Inport  Port=4
  Abs : Abs
  Constant : Constant  Value=1000
  Constant1 : Constant  Value=1000
  Constant2 : Constant  Value=100
  Divide1 : Product  Inputs=*/
  Gain2 : Gain  Gain=-1
  Integrator : Integrator
  Integrator1 : Integrator
  Product : Product  RndMeth=Zero
  Product1 : Product  RndMeth=Zero
  Product2 : Product  RndMeth=Zero
  Product5 : Product  Inputs=*/  RndMeth=Zero
  Subsystem3 : Subsystem
  Sum : Sum  Inputs=|+-
  Sum1 : Sum  Inputs=|+-
  Sum2 : Sum  Inputs=|+--
  k : Outport
  wires:
  Product5/1 -> k/1
  Subsystem3/1(Out1) -> Product5/2
  Gain2/1 -> Product5/1
  omega/1 -> Product/1
  Vx/1 -> Sum/1, Abs/1
  Product/1 -> Sum/2
  Sum/1 -> Sum1/2  "Vsx"
  Sum1/1 -> Product1/1, Integrator/1
  Integrator/1 -> Product2/1
  Product2/1 -> Sum2/2
  Product1/1 -> Sum2/3
  Integrator1/1 -> Sum1/1, Gain2/1  "Vsxstern"
  Sum2/1 -> Divide1/1
  Divide1/1 -> Integrator1/1
  Abs/1 -> Subsystem3/1(In1)
  Fx/1 -> Sum2/1
  Constant/1 -> Product1/2  "<dcx>"
  Constant1/1 -> Product2/2  "<kcx>"
  R/1 -> Product/2
  Constant2/1 -> Divide1/2

== system Model_Platform/Vehicle model/Drive_Train/4_Wheels_drive_train_and_Brake/RR/Alpha_Kappa_Selector2/alpha_calc ==
  Vy : Inport
  Vx : Inport  Port=2
  Ground : Ground
  Slip_angle_Calculation_From_Vx_and_Vy1 : Subsystem
  Terminator : Terminator
  front : Subsystem
  alpha : Outport
  wires:
  Slip_angle_Calculation_From_Vx_and_Vy1/1(Slip_Angle[deg]) -> alpha/1
  Ground/1 -> front/3(steering_angle)
  front/1(alpha) -> Terminator/1
  Vy/1 -> front/1(Vy), Slip_angle_Calculation_From_Vx_and_Vy1/2(Vy_CoG[m|s])
  Vx/1 -> front/2(Vx), Slip_angle_Calculation_From_Vx_and_Vy1/1(Vx_CoG[m|s])

== system Model_Platform/Vehicle model/Drive_Train/4_Wheels_drive_train_and_Brake/RR/Wheel dynamics/Friction ==
  omega_radPs : Inport
  Lookup Table : Lookup_n-D  NumberOfTableDimensions=1  BreakpointsForDimension1=omega_wheel  BeginIndexSearchUsingPreviousIndexResult=on  Table=Torque_lost_wheel  InputSameDT=on
  Product : Product  RndMeth=Zero
  Torque_friction : Outport
  wires:
  Lookup Table/1 -> Product/1
  Product/1 -> Torque_friction/1
  omega_radPs/1 -> Lookup Table/1, Product/2

== system Model_Platform/Vehicle model/Drive_Train/4_Wheels_drive_train_and_Brake/RR/Wheel dynamics/Subsystem ==
  Torque_Brake_Nm : Inport
  Omega_rad/s : Inport  Port=2
  Compare To Constant : simulink/Logic and Bit Operations/Compare To Constant  relop=>=  const=0.1  OutDataTypeStr=uint8
  Compare To Constant1 : simulink/Logic and Bit Operations/Compare To Constant  relop=<=  const=-0.1  OutDataTypeStr=uint8
  Data Type Conversion : DataTypeConversion
  Logical Operator : Logic  Operator=OR  AllPortsSameDT=off  OutDataTypeStr=boolean
  Product : Product  Inputs=3  RndMeth=Zero
  Rate Limiter1 : RateLimiter  SampleTimeMode=inherited
  Sign : Signum
  Torque_Brake_act_Nm : Outport
  wires:
  Torque_Brake_Nm/1 -> Product/1
  Omega_rad/s/1 -> Compare To Constant1/1, Compare To Constant/1, Sign/1
  Product/1 -> Torque_Brake_act_Nm/1
  Sign/1 -> Product/2
  Compare To Constant/1 -> Logical Operator/1
  Data Type Conversion/1 -> Rate Limiter1/1
  Logical Operator/1 -> Data Type Conversion/1
  Compare To Constant1/1 -> Logical Operator/2
  Rate Limiter1/1 -> Product/3

== system Model_Platform/Vehicle model/Vehicle dynamics/Vertical_Dyn./suspention_System/Rear_Right_Suspention/vertical_dynamics_tire ==
  note: z1
  note: F0
  note: U
  Force_Suspention : Inport
  Vertical_Displacement_Z0_Road : Inport  Port=2
  intial_force_form_mass : Inport  Port=3
  1/Mu : Gain  Gain=1/Para.VD.wheel_Mass.v
  Add1 : Sum  Inputs=++-
  Add2 : Sum  Inputs=+-
  Gain : Gain  Gain=Para.VD.Tire_Stifness.v
  Gain2 : Gain  Gain=Para.VD.Tire_Damping_Constant.v
  Integrator : Integrator
  Integrator1 : Integrator
  Relational Operator : RelationalOperator  Operator=>  OutDataTypeStr=boolean  ZeroCross=off  RndMeth=Nearest
  Saturation : Saturate  UpperLimit=Para.VD.Tire_intial_length.v-Para.VD.Tire_Lower_limit.v  LowerLimit=Para.VD.Tire_intial_length.v-Para.VD.Tire_Upper_limit.v
  Subtract2 : Sum  Inputs=+-
  Subtract3 : Sum  Inputs=+-
  Sum : Sum  Inputs=|++
  Switch : Switch
  Transfer Fcn : TransferFcn  Numerator=[1 0]  Denominator=[0.001 1]
  Transfer Fcn1 : TransferFcn  Numerator=[1 0]  Denominator=[0.001 1]
  Vertical_Displacement_Z1_Wheel : Outport
  Vertical_Velocity_Z1_Wheel : Outport  Port=2
  wires:
  Switch/1 -> Vertical_Displacement_Z1_Wheel/1, Transfer Fcn1/1
  Relational Operator/1 -> Switch/2
  Add2/1 -> Switch/1
  intial_force_form_mass/1 -> Sum/1
  Sum/1 -> Add1/1
  Gain/1 -> Sum/2
  Force_Suspention/1 -> Add1/3
  Vertical_Displacement_Z0_Road/1 -> Transfer Fcn/1, Subtract2/1, Add2/1
  Transfer Fcn/1 -> Subtract3/1
  Subtract2/1 -> Relational Operator/1, Saturation/1
  Saturation/1 -> Add2/2, Relational Operator/2, Gain/1
  Gain2/1 -> Add1/2
  Subtract3/1 -> Gain2/1
  Integrator1/1 -> Switch/3, Subtract2/2
  Integrator/1 -> Subtract3/2, Integrator1/1
  1/Mu/1 -> Integrator/1
  Add1/1 -> 1/Mu/1
  Transfer Fcn1/1 -> Vertical_Velocity_Z1_Wheel/1

== system Model_Platform/Vehicle model/Vehicle dynamics/Vertical_Dyn./suspention_System/Rear_left_Suspention/vertical_dynamics_tire ==
  note: z1
  note: F0
  note: U
  Force_Suspention : Inport
  Vertical_Displacement_Z0_Road : Inport  Port=2
  intial_force_form_mass : Inport  Port=3
  1/Mu : Gain  Gain=1/Para.VD.wheel_Mass.v
  Add1 : Sum  Inputs=++-
  Add2 : Sum  Inputs=+-
  Gain : Gain  Gain=Para.VD.Tire_Stifness.v
  Gain2 : Gain  Gain=Para.VD.Tire_Damping_Constant.v
  Integrator : Integrator
  Integrator1 : Integrator
  Relational Operator : RelationalOperator  Operator=>  OutDataTypeStr=boolean  ZeroCross=off  RndMeth=Nearest
  Saturation : Saturate  UpperLimit=Para.VD.Tire_intial_length.v-Para.VD.Tire_Lower_limit.v  LowerLimit=Para.VD.Tire_intial_length.v-Para.VD.Tire_Upper_limit.v
  Subtract2 : Sum  Inputs=+-
  Subtract3 : Sum  Inputs=+-
  Sum : Sum  Inputs=|++
  Switch : Switch
  Transfer Fcn : TransferFcn  Numerator=[1 0]  Denominator=[0.001 1]
  Transfer Fcn1 : TransferFcn  Numerator=[1 0]  Denominator=[0.001 1]
  Vertical_Displacement_Z1_Wheel : Outport
  Vertical_Velocity_Z1_Wheel : Outport  Port=2
  wires:
  Switch/1 -> Vertical_Displacement_Z1_Wheel/1, Transfer Fcn1/1
  Relational Operator/1 -> Switch/2
  Add2/1 -> Switch/1
  intial_force_form_mass/1 -> Sum/1
  Sum/1 -> Add1/1
  Gain/1 -> Sum/2
  Force_Suspention/1 -> Add1/3
  Vertical_Displacement_Z0_Road/1 -> Transfer Fcn/1, Subtract2/1, Add2/1
  Transfer Fcn/1 -> Subtract3/1
  Subtract2/1 -> Relational Operator/1, Saturation/1
  Saturation/1 -> Add2/2, Relational Operator/2, Gain/1
  Gain2/1 -> Add1/2
  Subtract3/1 -> Gain2/1
  Integrator1/1 -> Switch/3, Subtract2/2
  Integrator/1 -> Subtract3/2, Integrator1/1
  1/Mu/1 -> Integrator/1
  Add1/1 -> 1/Mu/1
  Transfer Fcn1/1 -> Vertical_Velocity_Z1_Wheel/1

== system Model_Platform/Vehicle model/Vehicle dynamics/Vertical_Dyn./suspention_System/front_left_Suspention/vertical_dynamics_tire ==
  note: z1
  note: F0
  note: U
  Force_Suspention : Inport
  Vertical_Displacement_Z0_Road : Inport  Port=2
  intial_force_form_mass : Inport  Port=3
  1/Mu : Gain  Gain=1/Para.VD.wheel_Mass.v
  Add1 : Sum  Inputs=++-
  Add2 : Sum  Inputs=+-
  Gain : Gain  Gain=Para.VD.Tire_Stifness.v
  Gain2 : Gain  Gain=Para.VD.Tire_Damping_Constant.v
  Integrator : Integrator
  Integrator1 : Integrator
  Relational Operator : RelationalOperator  Operator=>  OutDataTypeStr=boolean  ZeroCross=off  RndMeth=Nearest
  Saturation : Saturate  UpperLimit=Para.VD.Tire_intial_length.v-Para.VD.Tire_Lower_limit.v  LowerLimit=Para.VD.Tire_intial_length.v-Para.VD.Tire_Upper_limit.v
  Subtract2 : Sum  Inputs=+-
  Subtract3 : Sum  Inputs=+-
  Sum : Sum  Inputs=|++
  Switch : Switch
  Transfer Fcn : TransferFcn  Numerator=[1 0]  Denominator=[0.001 1]
  Transfer Fcn1 : TransferFcn  Numerator=[1 0]  Denominator=[0.001 1]
  Vertical_Displacement_Z1_Wheel : Outport
  Vertical_Velocity_Z1_Wheel : Outport  Port=2
  wires:
  Switch/1 -> Vertical_Displacement_Z1_Wheel/1, Transfer Fcn1/1
  Relational Operator/1 -> Switch/2
  Add2/1 -> Switch/1
  intial_force_form_mass/1 -> Sum/1
  Sum/1 -> Add1/1
  Gain/1 -> Sum/2
  Force_Suspention/1 -> Add1/3
  Vertical_Displacement_Z0_Road/1 -> Transfer Fcn/1, Subtract2/1, Add2/1
  Transfer Fcn/1 -> Subtract3/1
  Subtract2/1 -> Relational Operator/1, Saturation/1
  Saturation/1 -> Add2/2, Relational Operator/2, Gain/1
  Gain2/1 -> Add1/2
  Subtract3/1 -> Gain2/1
  Integrator1/1 -> Switch/3, Subtract2/2
  Integrator/1 -> Subtract3/2, Integrator1/1
  1/Mu/1 -> Integrator/1
  Add1/1 -> 1/Mu/1
  Transfer Fcn1/1 -> Vertical_Velocity_Z1_Wheel/1

== system Model_Platform/Vehicle model/Vehicle dynamics/Vertical_Dyn./suspention_System/front_right_Suspention/vertical_dynamics_tire ==
  note: z1
  note: F0
  note: U
  Force_Suspention : Inport
  Vertical_Displacement_Z0_Road : Inport  Port=2
  intial_force_form_mass : Inport  Port=3
  1/Mu : Gain  Gain=1/Para.VD.wheel_Mass.v
  Add1 : Sum  Inputs=++-
  Add2 : Sum  Inputs=+-
  Gain : Gain  Gain=Para.VD.Tire_Stifness.v
  Gain2 : Gain  Gain=Para.VD.Tire_Damping_Constant.v
  Integrator : Integrator
  Integrator1 : Integrator
  Relational Operator : RelationalOperator  Operator=>  OutDataTypeStr=boolean  ZeroCross=off  RndMeth=Nearest
  Saturation : Saturate  UpperLimit=Para.VD.Tire_intial_length.v-Para.VD.Tire_Lower_limit.v  LowerLimit=Para.VD.Tire_intial_length.v-Para.VD.Tire_Upper_limit.v
  Subtract2 : Sum  Inputs=+-
  Subtract3 : Sum  Inputs=+-
  Sum : Sum  Inputs=|++
  Switch : Switch
  Transfer Fcn : TransferFcn  Numerator=[1 0]  Denominator=[0.001 1]
  Transfer Fcn1 : TransferFcn  Numerator=[1 0]  Denominator=[0.001 1]
  Vertical_Displacement_Z1_Wheel : Outport
  Vertical_Velocity_Z1_Wheel : Outport  Port=2
  wires:
  Switch/1 -> Vertical_Displacement_Z1_Wheel/1, Transfer Fcn1/1
  Relational Operator/1 -> Switch/2
  Add2/1 -> Switch/1
  intial_force_form_mass/1 -> Sum/1
  Sum/1 -> Add1/1
  Gain/1 -> Sum/2
  Force_Suspention/1 -> Add1/3
  Vertical_Displacement_Z0_Road/1 -> Transfer Fcn/1, Subtract2/1, Add2/1
  Transfer Fcn/1 -> Subtract3/1
  Subtract2/1 -> Relational Operator/1, Saturation/1
  Saturation/1 -> Add2/2, Relational Operator/2, Gain/1
  Gain2/1 -> Add1/2
  Subtract3/1 -> Gain2/1
  Integrator1/1 -> Switch/3, Subtract2/2
  Integrator/1 -> Subtract3/2, Integrator1/1
  1/Mu/1 -> Integrator/1
  Add1/1 -> 1/Mu/1
  Transfer Fcn1/1 -> Vertical_Velocity_Z1_Wheel/1

== system Model_Platform/Vehicle model/Drive_Train/4_Wheels_drive_train_and_Brake/FL/Alpha_Kappa_Selector2/Dynamik Anteil2/Subsystem3 ==
  In1 : Inport
  Abs : Abs  SaturateOnIntegerOverflow=on
  In3_Switch : Constant
  Relational Operator : RelationalOperator  RndMeth=Nearest
  Switch : Switch  Threshold=1  SaturateOnIntegerOverflow=on
  Out1 : Outport
  wires:
  Switch/1 -> Out1/1
  Relational Operator/1 -> Switch/2
  In3_Switch/1 -> Switch/3, Relational Operator/2
  Abs/1 -> Relational Operator/1
  In1/1 -> Abs/1, Switch/1

== system Model_Platform/Vehicle model/Drive_Train/4_Wheels_drive_train_and_Brake/FL/Alpha_Kappa_Selector2/alpha_calc/Slip_angle_Calculation_From_Vx_and_Vy1 ==
  Vx_CoG[m|s] : Inport
  Vy_CoG[m|s] : Inport  Port=2
  Add : Sum
  Add2 : Sum
  Compare To Constant1 : simulink/Logic and Bit Operations/Compare To Constant  relop=>=  const=1  OutDataTypeStr=boolean
  Constant1 : Constant  Value=eps
  Data Type Conversion : DataTypeConversion
  Divide : Product  Inputs=*/
  Gain : Gain  Gain=180/pi
  Math Function : Math  Operator=square  SaturateOnIntegerOverflow=on
  Math Function1 : Math  Operator=square  SaturateOnIntegerOverflow=on
  Product1 : Product  Inputs=3
  Sign : Signum
  Sqrt : Sqrt  AlgorithmType=Newton-Raphson  SaturateOnIntegerOverflow=on
  Trigonometric Function1 : Trigonometry  Operator=atan
  Unary Minus1 : UnaryMinus
  Slip_Angle[deg] : Outport
  wires:
  Unary Minus1/1 -> Product1/3
  Sign/1 -> Unary Minus1/1
  Trigonometric Function1/1 -> Product1/1
  Constant1/1 -> Add2/2
  Add2/1 -> Divide/2
  Divide/1 -> Trigonometric Function1/1
  Sqrt/1 -> Compare To Constant1/1
  Add/1 -> Sqrt/1
  Math Function1/1 -> Add/2
  Math Function/1 -> Add/1
  Vx_CoG[m|s]/1 -> Add2/1, Math Function/1, Sign/1
  Vy_CoG[m|s]/1 -> Divide/1, Math Function1/1
  Compare To Constant1/1 -> Data Type Conversion/1
  Data Type Conversion/1 -> Product1/2
  Product1/1 -> Gain/1
  Gain/1 -> Slip_Angle[deg]/1
